simulink library "magnetorquer_lqr"  (R2016b)
settings: Solver=VariableStepAuto  StartTime=0.0  StopTime=10.0  RelTol=1e-3
undefined symbols (not defined in the file or in its folder): fsw_params
settings Model: Creator=sexymathemagician  LastModifiedBy=sexymathemagician

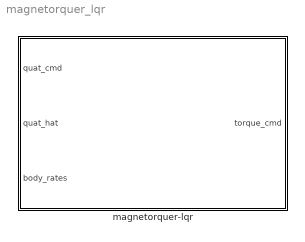
== system magnetorquer_lqr ==
  "magnetorquer-lqr " : Subsystem

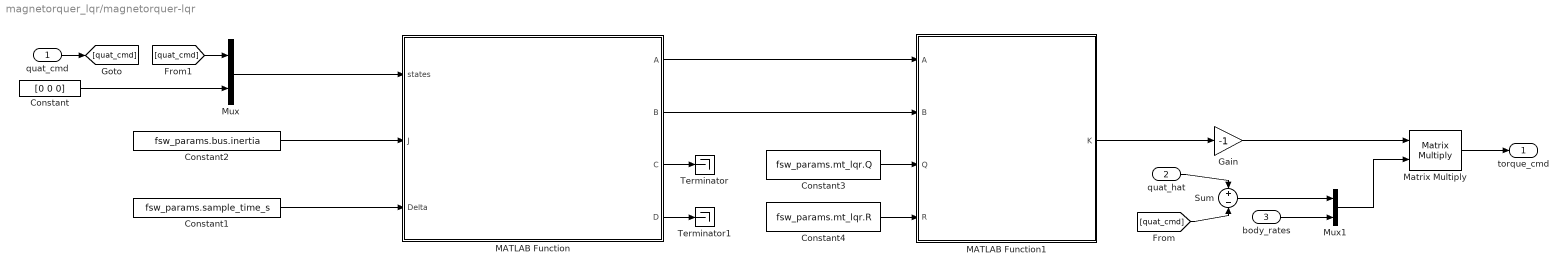
== system magnetorquer_lqr/magnetorquer-lqr  ==
  quat_cmd : Inport
  quat_hat : Inport  Port=2
  body_rates : Inport  Port=3
  Constant : Constant  Value=[0 0 0]
  Constant1 : Constant  Value=fsw_params.sample_time_s
  Constant2 : Constant  Value=fsw_params.bus.inertia
  Constant3 : Constant  Value=fsw_params.mt_lqr.Q
  Constant4 : Constant  Value=fsw_params.mt_lqr.R
  Gain : Gain  Gain=-1
  MATLAB Function : MATLAB Function  TreatAsAtomicUnit=on
  MATLAB Function1 : MATLAB Function  TreatAsAtomicUnit=on
  Matrix Multiply : Product  Multiplication=Matrix(*)
  Mux : Mux  Inputs=2
  Mux1 : Mux  Inputs=2
  Sum : Sum  Inputs=+-
  Terminator : Terminator
  Terminator1 : Terminator
  torque_cmd : Outport
  wires:
  Constant/1 -> Mux/2
  Mux/1 -> MATLAB Function/1(states)
  MATLAB Function/3(C) -> Terminator/1
  MATLAB Function/4(D) -> Terminator1/1
  Constant1/1 -> MATLAB Function/3(Delta)
  Constant2/1 -> MATLAB Function/2(J)
  MATLAB Function/1(A) -> MATLAB Function1/1(A)
  MATLAB Function/2(B) -> MATLAB Function1/2(B)
  Constant3/1 -> MATLAB Function1/3(Q)
  Constant4/1 -> MATLAB Function1/4(R)
  quat_cmd/1 -> [quat_cmd]
  [quat_cmd] -> Mux/1
  quat_hat/1 -> Sum/1
  [quat_cmd] -> Sum/2
  Sum/1 -> Mux1/1
  body_rates/1 -> Mux1/2
  MATLAB Function1/1(K) -> Gain/1
  Gain/1 -> Matrix Multiply/1
  Matrix Multiply/1 -> torque_cmd/1
  Mux1/1 -> Matrix Multiply/2

== matlab function magnetorquer_lqr/magnetorquer-lqr /MATLAB Function1 ==
  data: A input; K output; B input; Q input; R input
function K = lqr_command(A,B,Q,R)
%#codegen

[~,~,K] = care(A,B,Q,R); 

end

== matlab function magnetorquer_lqr/magnetorquer-lqr /MATLAB Function ==
  data: states input; A output; J input; Delta input; B output; C output; D output
function [A, B, C, D] = linearization(states, J, Delta)
%#codegen
q = states(1:4);
w = states(5:7);

XIq     = [ q(1) -q(2)  q(3);
           q(2)  q(1) -q(4);
          -q(3)  q(4)  q(1);
          -q(2) -q(3) -q(4) ];

XIw     = [  0   -w(1)  w(2)  w(1);
           w(1)   0   -w(3)  w(2);
          -w(2)  w(3)   0    w(3);
          -w(1) -w(2) -w(3)   0  ];

AA = [ 0.5*XIw 0.5*XIq;
       zeros(3,4) zeros(3,3) ];

J_inv = inv(J);
B = [zeros(4,3); J_inv];
A = AA;
C = eye(Nx);
D = zeros(7,3);

end
